simulink model "Simulation"  (R2025b)
settings: Solver=ode4  StartTime=0.0  StopTime=60  FixedStep=Ts  RelTol=1e-3
undefined symbols (not defined in the file or in its folder): A_SS_FD1, A_SS_FD3, A_zeta_f, A_zeta_tau, B_SS_FD1, B_SS_FD3, C_SS_FD1, C_SS_FD3, C_zeta_f, C_zeta_tau, D_SS_FD1, D_SS_FD3, eigs_NDO_force, eigs_NDO_torque, F1, F2, g_vec, inertia_factor, J, m, mass_factor, NDOB_force, NDOB_torque, period, radius, ReferenceTypeNumber, speed, Th_lower, Th_upper, Ts, Ts_hw, x0_FD1
libraries: simulink x9, dspstat3 x2
(part 2 of 2)

== matlab function Simulation/Fault Detection (FD) Module/Evaluator/MATLAB Function2 ==
  settings: updateMethod=DISCRETE  sampleTime=0.01
  data: raw_alarm input; confirmed_alarm output; current_time input; T_debounce parameter
function confirmed_alarm = debounce_logic(raw_alarm, current_time, T_debounce)
    % DEBOUNCE_LOGIC: Valida un allarme solo se rimane attivo per T_debounce secondi.
    
    % Definiamo le variabili "persistent". 
    % In Simulink, una variabile persistent ricorda il suo valore al ciclo 
    % di calcolo successivo (si comporta come la memoria di un flip-flop).
    persistent timer_start
    persistent is_timing
    
    % Inizializzazione: al tempo t=0, le variabili sono vuote
    if isempty(timer_start)
        timer_start = 0;       % Memoria del tempo in cui l'allarme è scattato
        is_timing = false;     % Flag: il cronometro sta girando?
    end
    
    % Di default, l'allarme confermato è sempre spento (0)
    confirmed_alarm = 0;
    
    % LOGICA DI VALUTAZIONE
    if raw_alarm == 1
        % L'errore grezzo ha superato la soglia!
        
        if ~is_timing
            % Se il cronometro era fermo, lo facciamo partire ORA
            timer_start = current_time;
            is_timing = true;
        end
        
        % Controlliamo da quanto tempo sta suonando l'allarme grezzo
        tempo_trascorso = current_time - timer_start;
        
        if tempo_trascorso >= T_debounce
            % Il tempo è scaduto! L'allarme è reale e confermato.
            confirmed_alarm = 1;
        end
        
    else
        % L'errore grezzo è tornato a 0 (sotto la soglia).
        % Potrebbe essere stato un falso allarme o il guasto è rientrato.
        % RESETTIAMO IL CRONOMETRO.
        is_timing = false;
        confirmed_alarm = 0;
    end
end

== matlab function Simulation/Fault Detection (FD) Module/Evaluator/MATLAB Function3 ==
  settings: updateMethod=DISCRETE  sampleTime=0.01
  data: raw_alarm input; confirmed_alarm output; current_time input; T_debounce parameter
function confirmed_alarm = debounce_logic(raw_alarm, current_time, T_debounce)
    % DEBOUNCE_LOGIC: Valida un allarme solo se rimane attivo per T_debounce secondi.
    
    % Definiamo le variabili "persistent". 
    % In Simulink, una variabile persistent ricorda il suo valore al ciclo 
    % di calcolo successivo (si comporta come la memoria di un flip-flop).
    persistent timer_start
    persistent is_timing
    
    % Inizializzazione: al tempo t=0, le variabili sono vuote
    if isempty(timer_start)
        timer_start = 0;       % Memoria del tempo in cui l'allarme è scattato
        is_timing = false;     % Flag: il cronometro sta girando?
    end
    
    % Di default, l'allarme confermato è sempre spento (0)
    confirmed_alarm = 0;
    
    % LOGICA DI VALUTAZIONE
    if raw_alarm == 1
        % L'errore grezzo ha superato la soglia!
        
        if ~is_timing
            % Se il cronometro era fermo, lo facciamo partire ORA
            timer_start = current_time;
            is_timing = true;
        end
        
        % Controlliamo da quanto tempo sta suonando l'allarme grezzo
        tempo_trascorso = current_time - timer_start;
        
        if tempo_trascorso >= T_debounce
            % Il tempo è scaduto! L'allarme è reale e confermato.
            confirmed_alarm = 1;
        end
        
    else
        % L'errore grezzo è tornato a 0 (sotto la soglia).
        % Potrebbe essere stato un falso allarme o il guasto è rientrato.
        % RESETTIAMO IL CRONOMETRO.
        is_timing = false;
        confirmed_alarm = 0;
    end
end

== matlab function Simulation/Fault Detection (FD) Module/Evaluator/r_gyro_norm ==
  data: r_vec input; r_norm output
function r_norm = fcn(r_vec)
    % Calcola la norma Euclidea del vettore 3x1
    r_norm = norm(r_vec);
end

== matlab function Simulation/Fault Detection (FD) Module/Evaluator/r_gps_norm ==
  data: r_vec input; r_norm output
function r_norm = fcn(r_vec)
    % Calcola la norma Euclidea del vettore 3x1
    r_norm = norm(r_vec);
end

== matlab function Simulation/Fault Detection (FD) Module/Evaluator/r_act_norm ==
  data: r_vec input; r_norm output
function r_norm = fcn(r_vec)
    % Calcola la norma Euclidea del vettore 3x1
    r_norm = norm(r_vec);
end

== matlab function Simulation/Fault Detection (FD) Module/Evaluator/MATLAB Function ==
  data: Fe_z input; alarm output; Th_upper parameter; Th_lower parameter
function alarm = Evaluator_Z(Fe_z, Th_upper, Th_lower)
%#codegen
% Questo Evaluator controlla se la stima della forza Z esce dalla 
% normale banda di tolleranza del vento per più di 0.5 secondi.

    % Parametri fissi
    sample_time = 0.001; 
    window_size = 0.5;   % Mezzo secondo di conferma

    % Memoria del timer
    persistent timer
    if isempty(timer)
        timer = 0;
    end
    
    % Controllo di sfondamento della soglia (sia in alto che in basso)
    if (Fe_z > Th_upper) || (Fe_z < Th_lower)
        timer = timer + sample_time;
    else
        timer = 0;
    end
    
    % Attivazione allarme
    if timer >= window_size
        alarm = 1;
    else
        alarm = 0;
    end
end

== matlab function Simulation/Algorithm to deploy/Controller/Subsystem/Force Observer (NDO) ==
  data: z input; pdot input; R input; u input; zdot output; Fe_E_hat output; Fe_E_dot_hat output; Fe_E_ddot_hat output; mask_F1 parameter; mask_g parameter; mask_m parameter; mask_C parameter; mask_A parameter; mask_AH parameter; mask_H parameter
function [zdot,Fe_E_hat,Fe_E_dot_hat,Fe_E_ddot_hat] = ForceNDO(z,pdot,R,u,mask_F1, mask_g, mask_m, mask_C, mask_A, mask_AH,mask_H)

% Constants
e3 = [0; 0; 1];

zetahat = z + mask_H*mask_m*pdot;
zdot = mask_AH*zetahat - mask_H*(mask_m*mask_g*e3 + R*mask_F1*u);
Fe_E_hat = mask_C*zetahat;
Fe_E_dot_hat = mask_C*mask_A*zetahat;
Fe_E_ddot_hat = mask_C*mask_A^2*zetahat;

end

== matlab function Simulation/Algorithm to deploy/Controller/Feedback linearization stage for standard multirotors/Dynamic Feedback Linearization ==
  data: fzdot input; fzddot output; fz input; p input; pdot input; omega input; R input; ulp input; ulyaw input; vp output; mask_m parameter; mask_g parameter; Fe_E_ddot_hat input; Mm_B_hat input; mask_Jinv parameter; mask_J parameter; vq output; vr output; mask_na parameter; rpy input; T3rd input; Tdot3rd input
function [fzddot,vp,vq,vr] = Control(fzdot,fz,p,pdot,omega,R,ulp,ulyaw,mask_m, mask_g,Fe_E_ddot_hat,Mm_B_hat,mask_Jinv, mask_J,mask_na, rpy,T3rd,Tdot3rd)

% Constants
e1 = [1; 0; 0];
e2 = [0; 1; 0];
e3 = [0; 0; 1];

% Wrappers for short code
m = mask_m;
g = mask_g;
J = mask_J;
Jinv = mask_Jinv;

% General Kinematics
omegae = R*omega;
zB = R*e3;
zBdot = cross(omegae,zB);

% Lie derivatives
gomega = -Jinv*cross(omega,J*omega);
ge = R*gomega;
gp = -2*fzdot*zBdot - fz*(cross(omegae,zBdot) + cross(ge,zB));

% Linearization actions
out = R'*(-gp - fz*cross(zB,R*Jinv*Mm_B_hat) - Fe_E_ddot_hat + m*ulp);
fzddot = -out(3);
vp = out(2)/fz;
vq = -out(1)/fz;

% % Small angle approximation
% vr = -(e3'*gomega) + ulyaw;

% No small angle approximation
vr = (-Tdot3rd*omega - T3rd*gomega - T3rd(1)*vp - T3rd(2)*vq - T3rd*Jinv*Mm_B_hat + ulyaw)/T3rd(3);

% CONTROL - Constant Yaw v1
if norm(fz)<1e-3
    fz = 1e-3;
    error('Upward lift force can not be null. Singular point.')
end

end


function vhat = skew(v)
    e1 = [1 0 0]';
    e2 = [0 1 0]';
    e3 = [0 0 1]';
    vhat = [cross(v,e1) cross(v,e2) cross(v,e3)];
end

== matlab function Simulation/Algorithm to deploy/Controller/Subsystem1/Force Observer (NDO) ==
  data: z input; omega input; u input; zdot output; Me_B_hat output; Me_B_dot_hat output; Me_B_ddot_hat output; mask_J parameter; mask_C parameter; mask_A parameter; mask_AH parameter; mask_H parameter; mask_F2 parameter
function [zdot,Me_B_hat,Me_B_dot_hat,Me_B_ddot_hat] = TorqueNDO(z,omega,u,mask_J, mask_C, mask_A, mask_AH,mask_H, mask_F2)

zetahat = z + mask_H*mask_J*omega;
zdot = mask_AH*zetahat - mask_H*(-cross(omega,mask_J*omega) + mask_F2*u);
Me_B_hat = mask_C*zetahat;
Me_B_dot_hat = mask_C*mask_A*zetahat;
Me_B_ddot_hat = mask_C*mask_A^2*zetahat;

end

== matlab function Simulation/Algorithm to deploy/Controller/MATLAB Function2 ==
  data: R input; rpy output
function rpy = fcn(R)

[rpy_new,~] = rotm2eul(R);
rpy = flip(rpy_new');

end

== matlab function Simulation/Algorithm to deploy/Controller/Feedback linearization stage for standard multirotors/MATLAB Function ==
  data: rpy input; Tdot3rd output; omega input
function Tdot3rd = getTdot(rpy,omega)
    % Calculate the time derivative of the kinematic coordinate tranformation
    % related to roll-pitch-yaw angles
    % T = getT(eta,omega), where eta = [phi; theta; psi] and omega = [p; q; r]
    % T = getT(phi,theta,psi,p,q,r)
    %
    % phi, theta, psi are, in order, roll, pitch and yaw angles.
    phi = rpy(1);
    theta = rpy(2);
    p = omega(1);
    q = omega(2);
    r = omega(3);
    Tdot3rd = [0,(cos(phi)*(p + r*cos(phi)*tan(theta) + q*sin(phi)*tan(theta)))/cos(theta) + (sin(phi)*sin(theta)*(q*cos(phi) - r*sin(phi)))/cos(theta)^2,(cos(phi)*sin(theta)*(q*cos(phi) - r*sin(phi)))/cos(theta)^2 - (sin(phi)*(p + r*cos(phi)*tan(theta) + q*sin(phi)*tan(theta)))/cos(theta)];
end

== matlab function Simulation/Algorithm to deploy/Controller/MATLAB Function ==
  data: rpy input; T3rd output
function T3rd = getT(rpy)
    phi = rpy(1);
    theta = rpy(2);
    
    T3rd = [0 sin(phi)/cos(theta) cos(phi)/cos(theta)];
end

== matlab function Simulation/Ground Control Station (GCS)/Tracking References ==
  data: t input; pr output; prdot output; prddot output; yaw output; speed parameter; period parameter; radius parameter; ReferenceTypeNumber input; yawdot output; yawddot output
function [pr,prdot,prddot,yaw,yawdot,yawddot] = RefGen(t, speed, period, radius, ReferenceTypeNumber)

% Extended references with derivatives
% prExtended = [pr prdot prddot] in R^{3x3}
% yawExtended = [yaw yawdot yawddot] in R^{1x3}

r = radius;
T = period;
v = speed;

if ReferenceTypeNumber == 0  % Origin

    prExtended = [NullWaveExtended(t); NullWaveExtended(t); NullWaveExtended(t)];
    yawExtended = NullWaveExtended(t);

elseif ReferenceTypeNumber == 1  % Constant speed in direction of xE

    prExtended = [speed*rampExtended(t); NullWaveExtended(t); NullWaveExtended(t)];
    yawExtended = NullWaveExtended(t);

elseif ReferenceTypeNumber == 2  % Constant speed in direction of yE

    prExtended = [NullWaveExtended(t); speed*rampExtended(t); NullWaveExtended(t)];
    yawExtended = NullWaveExtended(t);

elseif ReferenceTypeNumber == 3  % Constant speed in direction of -zE

    prExtended = [NullWaveExtended(t); NullWaveExtended(t); -speed*rampExtended(t)];
    yawExtended = NullWaveExtended(t);

elseif ReferenceTypeNumber == 4  % Ascending spiral
    
    pulsation = 2*pi/period;
    prExtended = [radius*CosineWaveExtended(t,pulsation)-radius*[1 0 0]; radius*SineWaveExtended(t,pulsation); -speed*rampExtended(t)];
    yawExtended = zeros(1,3);

    % omegayaw = 2*pi/5;
    % yawExtended = SineWaveExtended(t,omegayaw);

elseif ReferenceTypeNumber == 5  % Ascending 8-shape

    pulsation = 2*pi/period;
    prExtended = [radius*CosineWaveExtended(t,pulsation)-radius*[1 0 0]; 0.5*radius*SineWaveExtended(t,2*pulsation); -speed*rampExtended(t)];
    yawExtended = zeros(1,3);

elseif ReferenceTypeNumber == 6  % Square around e3

    prExtended = zeros(3,3);
    yawExtended = zeros(1,3);
    
    % L = 2*r;
    % t2 = mod(t,T);
    % pr = (4*L/T)*[ramp(t2)-ramp(t2-T/4)-ramp(t2-T/2)+ramp(t2-3*T/4); ramp(t2-T/4)-ramp(t2-T/2)-ramp(t2-3*T/4)+ramp(t2-T); -v*t];
    % psir = 0;
elseif ReferenceTypeNumber == 7

    prExtended = [SawtoothWaveExtended(t,20); NullWaveExtended(t); NullWaveExtended(t)];
    yawExtended = zeros(1,3);

elseif ReferenceTypeNumber == 8
    
    prExtended = [NullWaveExtended(t); NullWaveExtended(t); -SawtoothWave(t,20) 0 0];
    yawExtended = zeros(1,3);

elseif ReferenceTypeNumber == 9  % Descending spiral
    
    pulsation = 2*pi/period;
    prExtended = [radius*CosineWaveExtended(t,pulsation)-radius*[1 0 0]; 0.5*radius*SineWaveExtended(t,2*pulsation); (speed/2)*rampExtended(t)];
    yawExtended = zeros(1,3);

elseif ReferenceTypeNumber == 10  % Descending 8-shape

    pulsation = 2*pi/period;
    prExtended = [radius*CosineWaveExtended(t,pulsation)-radius*[1 0 0]; radius*SineWaveExtended(t,2*pulsation); (speed/2)*rampExtended(t)];
    yawExtended = zeros(1,3);

else
    error('ReferenceType non supported.')
    prExtended = zeros(3,3);
    yawExtended = zeros(1,3);
end

pr = prExtended(:,1);
prdot = prExtended(:,2);
prddot = prExtended(:,3);
yaw = yawExtended(1);
yawdot = yawExtended(2);
yawddot = yawExtended(3);

end
%%%%%%%%%%%%%%%%%%%%%%%%%%%%%%%%%%%
%         Basic signals           %
%%%%%%%%%%%%%%%%%%%%%%%%%%%%%%%%%%%
function u = NullWave(t)
    u = 0;
end
function u = step(t)
    if t >= 0
        u = 1;
    else
        u = 0;
    end
end
function u = ramp(t)
    u = t*step(t);
end
function u = SquareWave(t,T)
    t = mod(t,T);
    u = step(t)-step(t-T/2);
end
function u = SawtoothWave(t,T)
    t = mod(t,T);
    u = ramp(t)-2*ramp(t-T/2);
end
function u = SineWave(t,omega)
    u = sin(omega*t);
end
function u = CosineWave(t,omega)
    u = cos(omega*t);
end
%%%%%%%%%%%%%%%%%%%%%%%%%%%%%%%%%%%
%    Signals with derivatives     %
%%%%%%%%%%%%%%%%%%%%%%%%%%%%%%%%%%%
function uExtended = NullWaveExtended(t)
    uExtended = [0 0 0];
end
function uExtended = stepExtended(t)
    u = step(t);
    udot = 0;
    uddot = 0;
    uExtended = [u udot uddot];
end
function uExtended = rampExtended(t)
    u = ramp(t);
    udot = step(t);
    uddot = 0;
    uExtended = [u udot uddot];
end
function uExtended = SquareWaveExtended(t,T)
    t = mod(t,T);
    u = step(t)-step(t-T/2);
    udot = 0;
    uddot = 0;
    uExtended = [u udot uddot];
end
function uExtended = SawtoothWaveExtended(t,T)
    t = mod(t,T);
    u = ramp(t)-2*ramp(t-T/2);
    udot = step(t) - 2*step(t-T/2);
    uddot = 0;
    uExtended = [u udot uddot];
end
function uExtended = SineWaveExtended(t,omega)
    uExtended = [SineWave(t,omega) omega*CosineWave(t,omega) -(omega^2)*SineWave(t,omega)];
end
function uExtended = CosineWaveExtended(t,omega)
    uExtended = [CosineWave(t,omega) -omega*SineWave(t,omega) -(omega^2)*CosineWave(t,omega)];
end

== matlab function Simulation/Fault Detection (FD) Module/MATLAB Function ==
  data: omega_hat input; corr output
% Alternativa piu' semplice: usa i valori numerici diretti
function corr = Gyro_Correction(omega_hat)
    Jx = 0.0266;  Jy = 0.0266;  Jz = 0.0498;
    wx = omega_hat(1); wy = omega_hat(2); wz = omega_hat(3);
    cross_x = wy*(Jz*wz) - wz*(Jy*wy);
    cross_y = wz*(Jx*wx) - wx*(Jz*wz);
    cross_z = wx*(Jy*wy) - wy*(Jx*wx);
    corr = [-cross_x/Jx; -cross_y/Jy; -cross_z/Jz];
end

== matlab function Simulation/Algorithm to deploy/Controller/Linear internal controller for standard multirotors/Linear controllers ==
  data: fzdot input; ulp output; fz input; p input; pdot input; omega input; R input; rpy input; pr input; prdot input; prddot input; yawr input; yawrdot input; yawrddot input; int_errp input; ulyaw output; mask_m parameter; mask_g parameter; mask_k0 parameter; mask_k1 parameter; mask_k2 parameter; mask_k3 parameter; mask_k4 parameter; mask_chkPID parameter; Fe_E input; Fe_E_dot input; T3rd input
function [ulp,ulyaw] = LinearControl(fzdot,fz,p,pdot,omega,R,rpy,pr,prdot,prddot,yawr,yawrdot,yawrddot,int_errp,mask_m, mask_g,mask_k0, mask_k1, mask_k2, mask_k3, mask_k4,mask_chkPID,Fe_E,Fe_E_dot,T3rd)

% Constants
e1 = [1; 0; 0];
e2 = [0; 1; 0];
e3 = [0; 0; 1];

% Wrappers for short code
m = mask_m;
g = mask_g;
k0 = mask_k0;
k1 = mask_k1;
k2 = mask_k2;
k3 = mask_k3;
k4 = mask_k4;

% General Kinematics
omegae = R*omega;
zB = R*e3;
zBdot = cross(omegae,zB);

% %%%%%%%%%%%%%%%%%%%%%%%%%%%%%%%%%%%%%%%%%%%%%
% %       Linear position controller #1       %
% %%%%%%%%%%%%%%%%%%%%%%%%%%%%%%%%%%%%%%%%%%%%%
% Linear motion
prddddot = zeros(3,1);
prdddot = zeros(3,1);
pddot = (m*g*e3-fz*zB + Fe_E)/m;
pdddot = (-fzdot*zB-fz*zBdot + Fe_E_dot)/m;
if mask_chkPID == 1
    ulp = prddddot - k4*(pdddot-prdddot) - k3*(pddot-prddot) - k2*(pdot-prdot) - k1*(p-pr) - k0*int_errp;
else
    ulp = prddddot - k3*(pdddot-prdddot) - k2*(pddot-prddot) - k1*(pdot-prdot) - k0*(p-pr);
end

% %%%%%%%%%%%%%%%%%%%%%%%%%%%%%%%%%%%%%%%%%%%%%
% %          Linear yaw controller #1         %
% %%%%%%%%%%%%%%%%%%%%%%%%%%%%%%%%%%%%%%%%%%%%%
polyyaw = poly([-1 -2]);
k0yaw = polyyaw(3);
k1yaw = polyyaw(2);
yaw = rpy(3);

% Small angle approzimation
% ulyaw = + yawrddot - k1yaw*(e3'*omega-yawrdot) - k0yaw*(yaw-yawr);   

% No small angle approximation
ulyaw = + yawrddot - k1yaw*(T3rd*omega-yawrdot) - k0yaw*(yaw-yawr);

end
